simulink model "CodeSysModel"  (R2020b)
settings: Solver=FixedStepAuto  StartTime=0.0  StopTime=inf  FixedStep=2e-2  MaxStep=1e-4  RelTol=1e-3
model workspace (MAT data in the model file):
  sensor_carga = Simulink.Parameter
  sensor_carga.DataType = 'auto'
  sensor_carga.Dimensions = [0 0]
values from neighbouring files (symbols this model uses):
  bcx = 1000e3    (= 1000000)    [Datos_simulacion.m]
  bcy = 500e3    (= 500000)    [Datos_simulacion.m]
  beq_tc = (bv_c+beq_cel)/Rw^2    (= 27000)    [Datos_simulacion.m]
  beq_ti = (b_h+beq_iel)/Rd^2    (= 28800)    [Datos_simulacion.m]
  bw = 30e3    (= 30000)    [Datos_simulacion.m]
  g = 9.80665    [Datos_simulacion.m]
  i_c = 15    [Datos_simulacion.m]
  i_i = 30    [Datos_simulacion.m]
  Kcd = Meq_c*polo_c*n    (= 472500)    [Datos_simulacion.m]
  Kci = Kcp*polo_c/n    (= 1938936.66179)    [Datos_simulacion.m]
  Kcp = Kcd*polo_c    (= 1513396.48861)    [Datos_simulacion.m]
  Kcy = 1.3e9    (= 1300000000)    [Datos_simulacion.m]
  Kid = Kcp*polo_i/n    (= 1815537.84919)    [Datos_simulacion.m]
  Kii = Meq_i*polo_i*n    (= 360000)    [Datos_simulacion.m]
  Kip = Kcd*polo_i    (= 1417080.12441)    [Datos_simulacion.m]
  Kw = 1800e3    (= 1800000)    [Datos_simulacion.m]
  Meq_c = m_c+Jeq_c/Rw^2    (= 59008)    [Datos_simulacion.m]
  Meq_i = m_h+Jeq_i/Rd^2    (= 48014.2222222)    [Datos_simulacion.m]
  Rd = 0.75    [Datos_simulacion.m]
  Rw = 0.5    [Datos_simulacion.m]
  Tau = 1e-3    (= 0.001)    [Datos_simulacion.m]
libraries: simulink x2, fuzblock x1, pid_lib x1, dspswit3 x1
settings Model: PauseTimes=6  Creator=GoniR  LastModifiedBy=GoniR
settings SolverCC: ConcurrentTasks=on  ZeroCrossAlgorithm=Adaptive  AutoInsertRateTranBlk=on
settings DebuggingCC: MaskedZcDiagnostic=none  IgnoredZcDiagnostic=none
settings HardwareCC: ProdHWDeviceType=AMD->x86-64 (Windows64)
settings SFSimCC: SimTargetLang=C++
settings ConfigComp: PLC_TargetIDE=codesys23

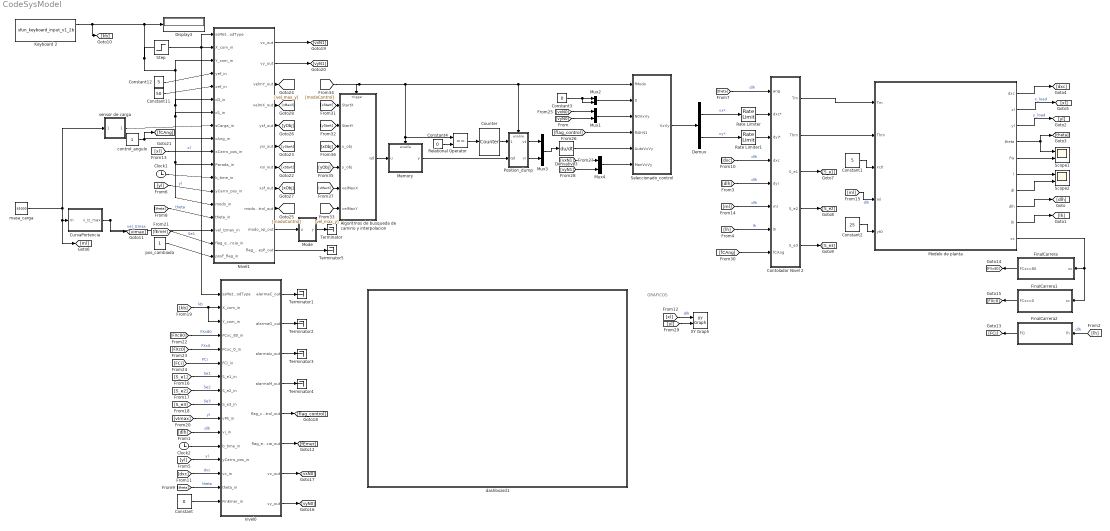
== system CodeSysModel ==
  note: GRAFICOS
  Algoritmos de busqueda de camino y interpolacion : Subsystem
  Clock1 : Clock
  Clock2 : Clock
  Constant : Constant  Value=0
  Constant1 : Constant  Value=5
  Constant11 : Constant  Value=50
  Constant12 : Constant  Value=5
  Constant2 : Constant  Value=25
  Constant3 : Constant  Value=0
  Constant4 : Constant  Value=0
  Contolador Nivel 2 : Subsystem
  Counter : dspswit3/Counter  Direction=Up  CountEvent=Free running  CounterSize=User defined  MaxCount=100000  InitialCount=0  Output=Count  HitValue=32  ResetInput=on  SamplesPerFrame=1  Ts=-1  CntDtype=double  HitDtype=Logical
  CurvaPortencia : MATLAB Function  TreatAsAtomicUnit=on
  Demux : Demux  Outputs=2
  Derivative3 : Derivative
  Display3 : Display
  FinalCarrera : Subsystem
  FinalCarrera1 : Subsystem
  FinalCarrera2 : Subsystem
  Keyboard 2 : M-S-Function  FunctionName=sfun_keyboard_input_v1_2b  mask(Keyboard Input){}
      mask help: Keyboard Input
      mask Display: fprintf('Keyboard');
  Memory : Subsystem
  Mode : MATLAB Function  TreatAsAtomicUnit=on
  Modelo de planta : Subsystem
  Mux{1..4} (4 alike) : Mux  Inputs=2
  Nivel1 : Subsystem  TreatAsAtomicUnit=on  SystemSampleTime=0.02
  Position_dump : Subsystem
  Rate Limiter : RateLimiter  RisingSlewLimit=2  FallingSlewLimit=-2  SampleTimeMode=inherited
  Rate Limiter1 : RateLimiter  RisingSlewLimit=2  FallingSlewLimit=-2  SampleTimeMode=inherited
  Relational Operator : RelationalOperator  Operator===  OutDataTypeStr=boolean  RndMeth=Simplest
  Scope1 : Scope  NumInputPorts=2
  Scope2 : Scope  NumInputPorts=2
  Seleccionado_control : Subsystem
  Step : Step  Time=0.01  SampleTime=0
  Terminator{,1..5} (6 alike) : Terminator
  XY Graph : simulink/Sinks/XY Graph  xmin=0  xmax=80  ymin=0  ymax=60  st=-1
  control_angulo : Constant
  dashboard1 : Subsystem
  masa_carga : Constant  Value=65000
  nivel0 : Subsystem  TreatAsAtomicUnit=on  SystemSampleTime=0.02
  pos_cambiada : Constant
  sensor de carga : Subsystem
  wires:
  Modelo de planta/2(xl) -> [xl]  "x_load"
  Modelo de planta/3(yl) -> [yl]  "y_load"
  Modelo de planta/7(dl) -> Scope2/2
  Modelo de planta/6(l) -> Scope2/1
  Modelo de planta/5(Fw) -> Scope1/2
  masa_carga/1 -> CurvaPortencia/1(m), [ml], sensor de carga/1(In1)
  Constant1/1 -> Modelo de planta/3(xc0)
  Constant2/1 -> Modelo de planta/5(yt0)
  Modelo de planta/4(theta) -> [theta], Scope1/1
  Memory/1(y) -> Position_dump/2(qd)
  Algoritmos de busqueda de camino y interpolacion/1(qd) -> Memory/1(u)
  Position_dump/2(vi) -> Mux3/2
  Demux/2 -> Rate Limiter1/1  "vy*"
  Demux/1 -> Rate Limiter/1  "vx*"
  Nivel1/10(modo_op_out) -> Mode/1(u)
  CurvaPortencia/1(v_Iz_max) -> Nivel1/16(vel_Izmax_in), [vImax]  "vel_Izmax"
  Mode/1(y) -> Terminator/1
  [modoControl] -> Algoritmos de busqueda de camino y interpolacion/Trigger, Relational Operator/1, Memory/Enable, Position_dump/Enable, Seleccionado_control/1(fModo)
  Nivel1/5(ysf_out) -> [yObj]
  Rate Limiter/1 -> Contolador Nivel 2/2(dxc*)
  Modelo de planta/1(dxc) -> [dxc]
  Modelo de planta/8(dlh) -> [dlh]
  Modelo de planta/9(lh) -> [lh]
  Contolador Nivel 2/1(Tm) -> Modelo de planta/1(Tm)
  Contolador Nivel 2/2(Thm) -> Modelo de planta/2(Thm)
  Rate Limiter1/1 -> Contolador Nivel 2/3(dyi*)
  Modelo de planta/10(xc) -> FinalCarrera1/1(xc), FinalCarrera/1(xc)
  Clock2/1 -> nivel0/12(b_time_in)
  nivel0/1(alarmaC_out) -> Terminator1/1
  nivel0/2(alarmaG_out) -> Terminator2/1
  nivel0/3(alarmaIz_out) -> Terminator3/1
  nivel0/4(alarmaM_out) -> Terminator4/1
  Mux3/1 -> Derivative3/1
  Constant/1 -> nivel0/16(FinEmer_in)
  nivel0/6(flag_emergencia_out) -> [fEmer]
  Constant3/1 -> Mux2/1, Mux2/2
  Position_dump/1(vt) -> Mux3/1
  Constant4/1 -> Relational Operator/2
  Relational Operator/1 -> Counter/1
  Counter/1 -> Position_dump/1(counter)
  [dlh] -> Contolador Nivel 2/5(dyi)  "dlh"
  [dlh] -> nivel0/11(vi_in)  "dlh"
  [lh] -> FinalCarrera2/1(lh)  "dlh"
  [lh] -> Contolador Nivel 2/7(lh)  "lh"
  [yl] -> nivel0/13(yCarro_pos_in)  "yl"
  [theta] -> Contolador Nivel 2/1(ang)  "dlh"
  [theta] -> nivel0/15(theta_in)  "theta"
  [dxc] -> Contolador Nivel 2/4(dxc)  "dlh"
  [dxc] -> nivel0/14(vc_in)  "dxc"
  [xl] -> XY Graph/1  "dlh"
  [xl] -> Nivel1/10(xCarro_pos_in)  "xl"
  [ml] -> Contolador Nivel 2/6(ml)  "dlh"
  [ml] -> Modelo de planta/4(ml)  "dlh"
  Contolador Nivel 2/3(S_e1) -> [S_e1]
  Contolador Nivel 2/4(S_e2) -> [S_e2]
  Contolador Nivel 2/5(S_e3) -> [S_e3]
  [S_e1] -> nivel0/7(S_e1_in)  "Se1"
  [S_e2] -> nivel0/8(S_e2_in)  "Se2"
  [S_e3] -> nivel0/9(S_e3_in)  "Se3"
  [kb] -> nivel0/3(Y_com_in), nivel0/2(X_com_in)  "kb"
  [vImax] -> nivel0/10(vMi_in)  "yl"
  FinalCarrera2/1(FCi) -> [FCi]
  FinalCarrera1/1(FCxc<0) -> [FXc0]
  FinalCarrera/1(FCxc>80) -> [FXc80]
  [FCi] -> nivel0/6(FCi_in)  "FCi"
  [FXc0] -> nivel0/5(FCxc_0_in)  "FXc0"
  [FXc80] -> nivel0/4(FCxc_80_in)  "FXc80"
  nivel0/8(vy_out) -> [vyN0]
  nivel0/7(vx_out) -> [vxN0]
  [vyN0] -> Mux1/2
  [vxN0] -> Mux1/1
  nivel0/5(flag_control_out) -> [flag_control]
  Nivel1/1(vx_out) -> [vxN1]
  Nivel1/2(vy_out) -> [vyN1]
  [vxN1] -> Mux4/1
  [vyN1] -> Mux4/2
  Mux2/1 -> Seleccionado_control/2(0)
  Mux1/1 -> Seleccionado_control/3(N0VxVy)
  [flag_control] -> Seleccionado_control/4(fN0-N1)
  Derivative3/1 -> Seleccionado_control/5(AutoVxVy)
  Mux4/1 -> Seleccionado_control/6(ManVxVy)
  Seleccionado_control/1(VxVy) -> Demux/1
  [yl] -> XY Graph/2
  Nivel1/11(flag_disDesP_out) -> Terminator5/1
  [fCAng] -> Contolador Nivel 2/8(fCAng)
  [yl] -> Nivel1/13(yCarro_pos_in)  "yl"
  [theta] -> Nivel1/15(theta_in)  "theta"
  [fEmer] -> Nivel1/17(flag_emergencia_in)  "Se1"
  Keyboard 2/1 -> Display3/1, Nivel1/2(X_com_in), Nivel1/3(Y_com_in), Nivel1/14(modo_in), Nivel1/11(Parada_in), Nivel1/7(cS_in), Nivel1/6(cD_in), [kb]
  Step/1 -> Nivel1/1(ssMethodType), nivel0/1(ssMethodType)
  Constant12/1 -> Nivel1/4(yef_in)
  Constant11/1 -> Nivel1/5(xef_in)
  sensor de carga/1(sCarga_in) -> Nivel1/8(sCarga_in)
  control_angulo/1 -> Nivel1/9(cAng_in), [fCAng]
  Clock1/1 -> Nivel1/12(b_time_in)
  pos_cambiada/1 -> Nivel1/18(posF_flag_in)
  Nivel1/7(xsi_out) -> [xStart]
  [xStart] -> Algoritmos de busqueda de camino y interpolacion/1(StartX)
  Nivel1/6(ysi_out) -> [yStart]
  [yStart] -> Algoritmos de busqueda de camino y interpolacion/2(StartY)
  [vel_max_y] -> Algoritmos de busqueda de camino y interpolacion/6(velMaxY)
  Nivel1/3(velmY_out) -> [vel_max_y]
  Nivel1/9(modo_de_control_out) -> [modoControl]
  [yObj] -> Algoritmos de busqueda de camino y interpolacion/4(y_obj)
  Nivel1/8(xsf_out) -> [xObj]
  [xObj] -> Algoritmos de busqueda de camino y interpolacion/3(x_obj)
  Nivel1/4(velmX_out) -> [vMaxX]
  [vMaxX] -> Algoritmos de busqueda de camino y interpolacion/5(velMaxX)

== system CodeSysModel/Algoritmos de busqueda de camino y interpolacion ==
  StartX : Inport
  StartY : Inport  Port=2
  x_obj : Inport  Port=3
  y_obj : Inport  Port=4
  velMaxX : Inport  Port=5
  velMaxY : Inport  Port=6
  Trigger : TriggerPort  VariantControl=Variant  PortDimensions=1
  Astart : MATLAB Function  TreatAsAtomicUnit=on
  Interpolador : MATLAB Function  TreatAsAtomicUnit=on
  qd : Outport
  wires:
  StartX/1 -> Astart/1(StartX)
  y_obj/1 -> Astart/4(y_obj)
  x_obj/1 -> Astart/3(x_obj)
  StartY/1 -> Astart/2(StartY)
  Astart/1(OptimalPath2) -> Interpolador/1(wayPoints)
  velMaxX/1 -> Interpolador/2(velMaxX)
  velMaxY/1 -> Interpolador/3(velMaxY)
  Interpolador/1(q) -> qd/1

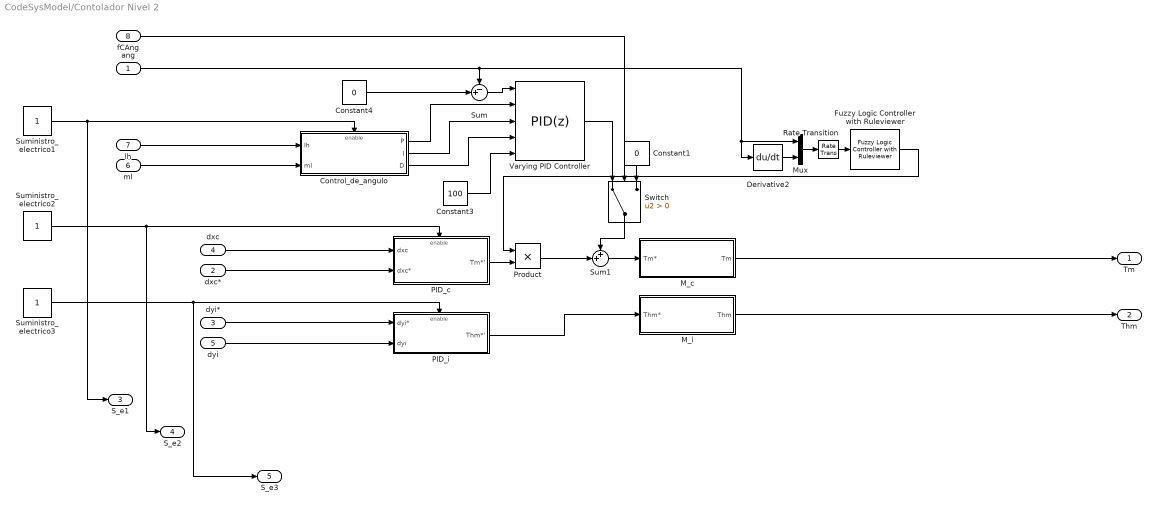
== system CodeSysModel/Contolador Nivel 2 ==
  ang : Inport
  dxc* : Inport  Port=2
  dyi* : Inport  Port=3
  dxc : Inport  Port=4
  dyi : Inport  Port=5
  ml : Inport  Port=6
  lh : Inport  Port=7
  fCAng : Inport  Port=8
  Constant1 : Constant  Value=0
  Constant3 : Constant  Value=100
  Constant4 : Constant  Value=0
  Control_de_angulo : Subsystem
  Derivative2 : Derivative
  Fuzzy Logic Controller with Ruleviewer : fuzblock/Fuzzy Logic  Controller  with Ruleviewer  fismatrix=Control2  Ts=0.5
  M_c : Subsystem
  M_i : Subsystem
  Mux : Mux  Inputs=2
  PID_c : Subsystem
  PID_i : Subsystem
  Product : Product
  Rate Transition : RateTransition  OutPortSampleTime=0.02
  Sum : Sum  Inputs=-+|
  Sum1 : Sum  Inputs=++|
  Suministro_electrico1 : Constant
  Suministro_electrico2 : Constant
  Suministro_electrico3 : Constant
  Switch : Switch  Criteria=u2 > Threshold
  Varying PID Controller : pid_lib/PID Controller  Controller=PID  Form=Parallel  TimeDomain=Discrete-time  UseExternalTs=off  SampleTime=0.02  IntegratorMethod=Forward Euler  FilterMethod=Forward Euler  ControllerParametersSource=external  P=1  I=1  D=0  UseFilter=on  N=100  TunerSelectOption=Transfer Function Based (PID Tuner App)  InitialConditionSource=internal  InitialConditionForIntegrator=0  InitialConditionForFilter=0  DifferentiatorICPrevScaledInput=0  ExternalReset=none  TrackingMode=off  Kt=1  LimitOutput=off  SatLimitsSource=internal  UpperSaturationLimit=inf  LowerSaturationLimit=-inf  LinearizeAsGain=on  AntiWindupMode=none  Kb=1  POutMin=[]  POutMax=[]  IOutMin=[]  IOutMax=[]  DOutMin=[]  DOutMax=[]  NOutMin=[]  NOutMax=[]  SumOutMin=[]  SumOutMax=[]  SaturationOutMin=[]  SaturationOutMax=[]  PParamMin=[]  PParamMax=[]  IParamMin=[]  IParamMax=[]  DParamMin=[]  DParamMax=[]  NParamMin=[]  NParamMax=[]  KbParamMin=[]  KbParamMax=[]  KtParamMin=[]  KtParamMax=[]  KbOutMin=[]  KbOutMax=[]  KtOutMin=[]  KtOutMax=[]  IntegratorOutMin=[]  IntegratorOutMax=[]  FilterOutMin=[]  FilterOutMax=[]  SumI1OutMin=[]  SumI1OutMax=[]  SumI2OutMin=[]  SumI2OutMax=[]  SumI3OutMin=[]  SumI3OutMax=[]  SumI4OutMin=[]  SumI4OutMax=[]  SumDOutMin=[]  SumDOutMax=[]  DifferentiatorOutMin=[]  DifferentiatorOutMax=[]  FilterDiffOutCoefMin=[]  FilterDiffOutCoefMax=[]  ReciprocalOutMin=[]  ReciprocalOutMax=[]  SumDenOutMin=[]  SumDenOutMax=[]  SumNumOutMin=[]  SumNumOutMax=[]  DivideOutMin=[]  DivideOutMax=[]  UdiffTsProdOutMin=[]  UdiffTsProdOutMax=[]  NTsProdOutMin=[]  NTsProdOutMax=[]  UintegralTsProdOutMin=[]  UintegralTsProdOutMax=[]  UngainTsProdOutMin=[]  UngainTsProdOutMax=[]  IntegratorContinuousStateAttributes=''  IntegratorStateMustResolveToSignalObject=off  IntegratorRTWStateStorageClass=Auto  FilterContinuousStateAttributes=''  FilterStateMustResolveToSignalObject=off  FilterRTWStateStorageClass=Auto  ParallelPVariant=ExternalParameters  IdealPVariant=Disabled  IVariant=ExternalParameters  DVariant=ExternalParameters  IntegratorVariant=Discrete  SatVariant=Disabled  AWVariant=Passthrough  PCopyVariant=Disabled  TRVariant=Disabled  FdbkBlocksVariant=Forward  IdealPFdbkVariant=Disabled  SatFdbkVariant=Disabled  DerivativeFilterVariant=ForwardEulerFilter  NVariant=ExternalParameters  NCopyVariant=Disabled  FilterICVariant=InternalICsFilter  IntegratorICVariant=InternalICs  ExternalResetVariant=Disabled  TRSumVariant=Passthrough  SumFdbkVariant=Disabled  SumVariant=Sum_PID  TsampFilterVariant=InternalTs  TsampNgainVariant=Passthrough  TsampIntegralVariant=Passthrough  ExternalSaturationOutDataTypeStr=Inherit: Same as second input
  Tm : Outport
  Thm : Outport  Port=2
  S_e1 : Outport  Port=3
  S_e2 : Outport  Port=4
  S_e3 : Outport  Port=5
  wires:
  Constant3/1 -> Varying PID Controller/5
  Fuzzy Logic Controller with Ruleviewer/1 -> Product/1
  Rate Transition/1 -> Fuzzy Logic Controller with Ruleviewer/1
  M_i/1(Thm) -> Thm/1
  ang/1 -> Derivative2/1, Mux/1, Sum/1
  Constant4/1 -> Sum/2
  Control_de_angulo/1(P) -> Varying PID Controller/2
  PID_i/1(Thm*') -> M_i/1(Thm*)
  Sum/1 -> Varying PID Controller/1
  Control_de_angulo/3(D) -> Varying PID Controller/4
  Product/1 -> Sum1/2
  Control_de_angulo/2(I) -> Varying PID Controller/3
  ml/1 -> Control_de_angulo/2(ml)
  Mux/1 -> Rate Transition/1
  PID_c/1(Tm*') -> Product/2
  Sum1/1 -> M_c/1(Tm*)
  M_c/1(Tm) -> Tm/1
  dxc*/1 -> PID_c/2(dxc*)
  lh/1 -> Control_de_angulo/1(lh)
  dyi*/1 -> PID_i/1(dyi*)
  dxc/1 -> PID_c/1(dxc)
  dyi/1 -> PID_i/2(dyi)
  Derivative2/1 -> Mux/2
  Suministro_electrico1/1 -> S_e1/1, Control_de_angulo/Enable
  Suministro_electrico3/1 -> PID_i/Enable, S_e3/1
  Suministro_electrico2/1 -> S_e2/1, PID_c/Enable
  Switch/1 -> Sum1/1
  fCAng/1 -> Switch/2
  Constant1/1 -> Switch/3
  Varying PID Controller/1 -> Switch/1

== system CodeSysModel/FinalCarrera ==
  xc : Inport
  Constant : Constant
  Constant1 : Constant  Value=0
  Switch : Switch  Criteria=u2 > Threshold  Threshold=80
  FCxc>80 : Outport
  wires:
  Constant/1 -> Switch/1
  Constant1/1 -> Switch/3
  Switch/1 -> FCxc>80/1
  xc/1 -> Switch/2

== system CodeSysModel/FinalCarrera1 ==
  xc : Inport
  Constant : Constant
  Constant1 : Constant  Value=0
  Gain : Gain  Gain=-1
  Switch : Switch  Criteria=u2 > Threshold
  FCxc<0 : Outport
  wires:
  Constant/1 -> Switch/1
  Constant1/1 -> Switch/3
  Switch/1 -> FCxc<0/1
  xc/1 -> Gain/1
  Gain/1 -> Switch/2

== system CodeSysModel/FinalCarrera2 ==
  lh : Inport
  Constant : Constant
  Constant1 : Constant  Value=0
  Gain : Gain  Gain=-1
  Switch : Switch
  FCi : Outport
  wires:
  Constant/1 -> Switch/1
  Constant1/1 -> Switch/3
  Switch/1 -> FCi/1
  lh/1 -> Gain/1
  Gain/1 -> Switch/2

== system CodeSysModel/Memory ==
  u : Inport
  Enable : EnablePort
  y : Outport
  wires:
  u/1 -> y/1

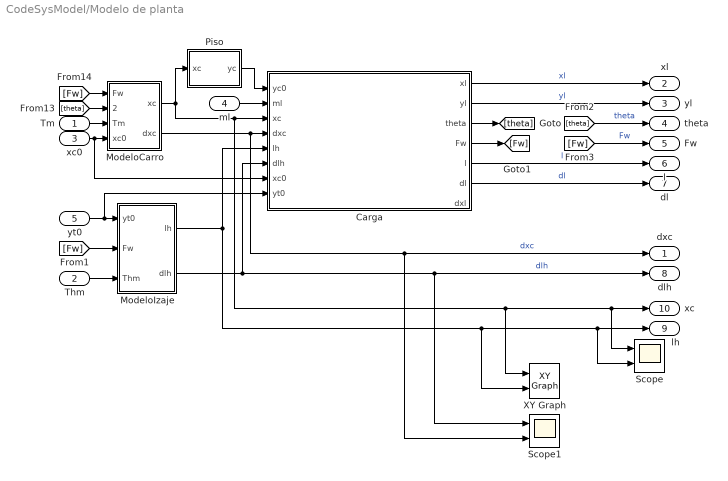
== system CodeSysModel/Modelo de planta ==
  Tm : Inport
  Thm : Inport  Port=2
  xc0 : Inport  Port=3
  ml : Inport  Port=4
  yt0 : Inport  Port=5
  Carga : Subsystem
  ModeloCarro : Subsystem
  ModeloIzaje : Subsystem
  Piso : Subsystem
  Scope : Scope  NumInputPorts=2
  Scope1 : Scope  NumInputPorts=2
  XY Graph : simulink/Sinks/XY Graph  xmin=0  xmax=80  ymin=0  ymax=60  st=-1
  dxc : Outport
  xl : Outport  Port=2
  yl : Outport  Port=3
  theta : Outport  Port=4
  Fw : Outport  Port=5
  l : Outport  Port=6
  dl : Outport  Port=7
  dlh : Outport  Port=8
  lh : Outport  Port=9
  xc : Outport  Port=10
  wires:
  ModeloCarro/1(xc) -> XY Graph/1, Scope/1, xc/1, Carga/3(xc), Piso/1(xc)
  ModeloCarro/2(dxc) -> Scope1/2, dxc/1, Carga/4(dxc)  "dxc"
  ModeloIzaje/1(lh) -> XY Graph/2, Scope/2, lh/1, Carga/5(lh)
  ModeloIzaje/2(dlh) -> Carga/6(dlh), Scope1/1, dlh/1  "dlh"
  Carga/4(Fw) -> [Fw]
  [Fw] -> ModeloCarro/1(Fw)
  [Fw] -> ModeloIzaje/2(Fw)
  Carga/3(theta) -> [theta]
  [theta] -> ModeloCarro/2(theta)
  Carga/1(xl) -> xl/1  "xl"
  Carga/2(yl) -> yl/1  "yl"
  Carga/5(l) -> l/1  "l"
  Carga/6(dl) -> dl/1  "dl"
  [theta] -> theta/1  "theta"
  [Fw] -> Fw/1  "Fw"
  ml/1 -> Carga/2(ml)
  Thm/1 -> ModeloIzaje/3(Thm)
  Tm/1 -> ModeloCarro/3(Tm)
  Piso/1(yc) -> Carga/1(yc0)
  yt0/1 -> Carga/8(yt0), ModeloIzaje/1(yt0)
  xc0/1 -> Carga/7(xc0), ModeloCarro/4(xc0)

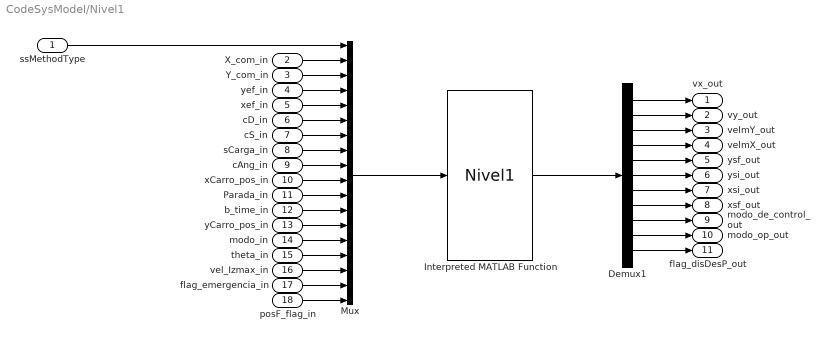
== system CodeSysModel/Nivel1 ==
  ssMethodType : Inport
  X_com_in : Inport  Port=2
  Y_com_in : Inport  Port=3
  yef_in : Inport  Port=4
  xef_in : Inport  Port=5
  cD_in : Inport  Port=6
  cS_in : Inport  Port=7
  sCarga_in : Inport  Port=8
  cAng_in : Inport  Port=9
  xCarro_pos_in : Inport  Port=10
  Parada_in : Inport  Port=11
  b_time_in : Inport  Port=12
  yCarro_pos_in : Inport  Port=13
  modo_in : Inport  Port=14
  theta_in : Inport  Port=15
  vel_Izmax_in : Inport  Port=16
  flag_emergencia_in : Inport  Port=17
  posF_flag_in : Inport  Port=18
  Demux1 : Demux  Outputs=11
  Interpreted MATLAB Function : MATLABFcn  MATLABFcn=Nivel1  OutputDimensions=11  Output1D=off
  Mux : Mux  Inputs=18
  vx_out : Outport
  vy_out : Outport  Port=2
  velmY_out : Outport  Port=3
  velmX_out : Outport  Port=4
  ysf_out : Outport  Port=5
  ysi_out : Outport  Port=6
  xsi_out : Outport  Port=7
  xsf_out : Outport  Port=8
  modo_de_control_out : Outport  Port=9
  modo_op_out : Outport  Port=10
  flag_disDesP_out : Outport  Port=11
  wires:
  Interpreted MATLAB Function/1 -> Demux1/1
  ssMethodType/1 -> Mux/1
  X_com_in/1 -> Mux/2
  Y_com_in/1 -> Mux/3
  yef_in/1 -> Mux/4
  xef_in/1 -> Mux/5
  cD_in/1 -> Mux/6
  cS_in/1 -> Mux/7
  sCarga_in/1 -> Mux/8
  cAng_in/1 -> Mux/9
  xCarro_pos_in/1 -> Mux/10
  Parada_in/1 -> Mux/11
  b_time_in/1 -> Mux/12
  yCarro_pos_in/1 -> Mux/13
  modo_in/1 -> Mux/14
  theta_in/1 -> Mux/15
  vel_Izmax_in/1 -> Mux/16
  flag_emergencia_in/1 -> Mux/17
  posF_flag_in/1 -> Mux/18
  Demux1/1 -> vx_out/1
  Demux1/2 -> vy_out/1
  Demux1/3 -> velmY_out/1
  Demux1/4 -> velmX_out/1
  Demux1/5 -> ysf_out/1
  Demux1/6 -> ysi_out/1
  Demux1/7 -> xsi_out/1
  Demux1/8 -> xsf_out/1
  Demux1/9 -> modo_de_control_out/1
  Demux1/10 -> modo_op_out/1
  Demux1/11 -> flag_disDesP_out/1
  Mux/1 -> Interpreted MATLAB Function/1

== system CodeSysModel/Position_dump ==
  counter : Inport
  qd : Inport  Port=2
  Enable : EnablePort  PropagateVarSize=During execution
  MATLAB Function : MATLAB Function  TreatAsAtomicUnit=on
  Rate Transition : RateTransition
  Scope1 : Scope
  vt : Outport
  vi : Outport  Port=2
  wires:
  MATLAB Function/1(vt) -> vt/1
  MATLAB Function/2(vi) -> vi/1
  qd/1 -> MATLAB Function/1(qd)
  Rate Transition/1 -> Scope1/1, MATLAB Function/2(cont_i)
  counter/1 -> Rate Transition/1

== system CodeSysModel/Seleccionado_control ==
  fModo : Inport
  0 : Inport  Port=2
  N0VxVy : Inport  Port=3
  fN0-N1 : Inport  Port=4
  AutoVxVy : Inport  Port=5
  ManVxVy : Inport  Port=6
  AutoOn/Off : Switch  Criteria=u2 > Threshold
  M_o_A : Switch  Criteria=u2 > Threshold
  N0_o_N1 : Switch  Criteria=u2 > Threshold
  VxVy : Outport
  wires:
  AutoOn/Off/1 -> M_o_A/1
  N0_o_N1/1 -> VxVy/1
  M_o_A/1 -> N0_o_N1/3
  ManVxVy/1 -> M_o_A/3
  AutoVxVy/1 -> AutoOn/Off/1
  fModo/1 -> AutoOn/Off/2, M_o_A/2
  0/1 -> AutoOn/Off/3
  fN0-N1/1 -> N0_o_N1/2
  N0VxVy/1 -> N0_o_N1/1

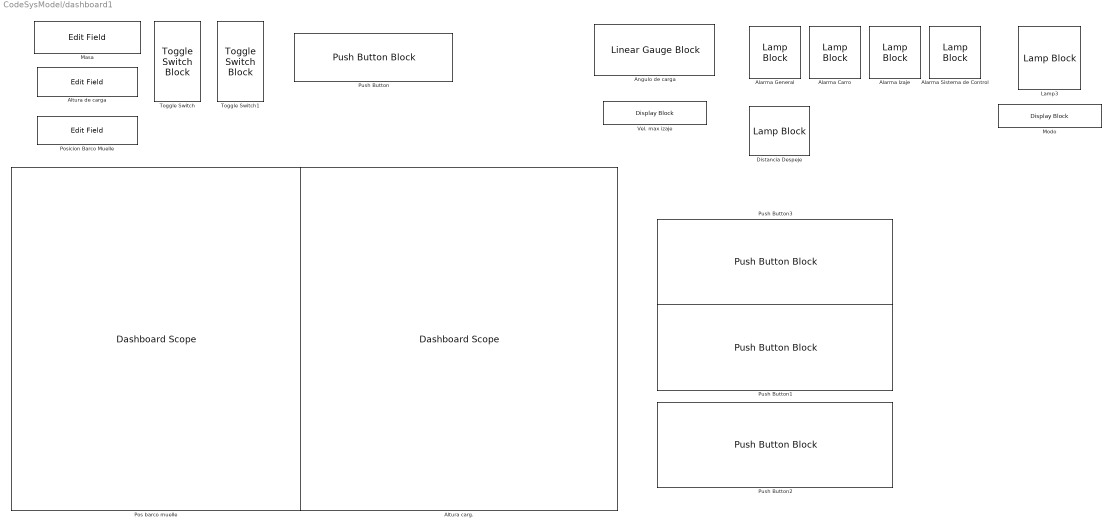
== system CodeSysModel/dashboard1 ==
  Alarma Carro : LampBlock
  Alarma General : LampBlock
  Alarma Izaje : LampBlock
  Alarma Sistema de Control : LampBlock
  Altura carg. : DashboardScope
  Altura de carga : EditField  LabelPosition=Hide  ShowInitialText=on  Alignment=Center
  Angulo de carga : LinearGaugeBlock  LabelPosition=Hide  ScaleMin=-0.15  ScaleMax=0.15
  Distancia Despeje : LampBlock
  Lamp3 : LampBlock  LabelPosition=Bottom
  Masa : EditField  LabelPosition=Hide  ShowInitialText=on  Alignment=Center
  Modo : DisplayBlock  LabelPosition=Hide  Format=short  Transparency=1
  Pos barco muelle : DashboardScope
  Posicion Barco Muelle : EditField  LabelPosition=Hide  ShowInitialText=on  Alignment=Center
  Push Button : PushButtonBlock  ButtonText=Fin Emergencia
  Push Button1 : PushButtonBlock  ButtonText=Falla Microcontrolador1  OnValue=0
  Push Button2 : PushButtonBlock  ButtonText=Falla Microcontrolador3  OnValue=0
  Push Button3 : PushButtonBlock  ButtonText=Falla Microcontrolador2  OnValue=0
  Toggle Switch : ToggleSwitchBlock
      settings: Values={{'Off', 'On'}, [0 1]}
  Toggle Switch1 : ToggleSwitchBlock
      settings: Values={{'Sin Cambiar', 'Cambiada'}, [0 1]}
  Vel. max izaje : DisplayBlock  LabelPosition=Hide  Format=short  Transparency=1

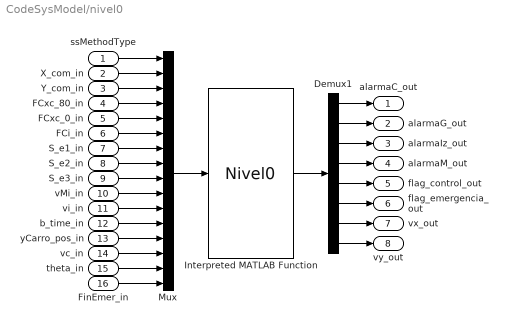
== system CodeSysModel/nivel0 ==
  ssMethodType : Inport
  X_com_in : Inport  Port=2
  Y_com_in : Inport  Port=3
  FCxc_80_in : Inport  Port=4
  FCxc_0_in : Inport  Port=5
  FCi_in : Inport  Port=6
  S_e1_in : Inport  Port=7
  S_e2_in : Inport  Port=8
  S_e3_in : Inport  Port=9
  vMi_in : Inport  Port=10
  vi_in : Inport  Port=11
  b_time_in : Inport  Port=12
  yCarro_pos_in : Inport  Port=13
  vc_in : Inport  Port=14
  theta_in : Inport  Port=15
  FinEmer_in : Inport  Port=16
  Demux1 : Demux  Outputs=8
  Interpreted MATLAB Function : MATLABFcn  MATLABFcn=Nivel0  OutputDimensions=8  Output1D=off
  Mux : Mux  Inputs=16
  alarmaC_out : Outport
  alarmaG_out : Outport  Port=2
  alarmaIz_out : Outport  Port=3
  alarmaM_out : Outport  Port=4
  flag_control_out : Outport  Port=5
  flag_emergencia_out : Outport  Port=6
  vx_out : Outport  Port=7
  vy_out : Outport  Port=8
  wires:
  Interpreted MATLAB Function/1 -> Demux1/1
  ssMethodType/1 -> Mux/1
  X_com_in/1 -> Mux/2
  Y_com_in/1 -> Mux/3
  FCxc_80_in/1 -> Mux/4
  FCxc_0_in/1 -> Mux/5
  FCi_in/1 -> Mux/6
  S_e1_in/1 -> Mux/7
  S_e2_in/1 -> Mux/8
  S_e3_in/1 -> Mux/9
  vMi_in/1 -> Mux/10
  vi_in/1 -> Mux/11
  b_time_in/1 -> Mux/12
  yCarro_pos_in/1 -> Mux/13
  vc_in/1 -> Mux/14
  theta_in/1 -> Mux/15
  FinEmer_in/1 -> Mux/16
  Demux1/1 -> alarmaC_out/1
  Demux1/2 -> alarmaG_out/1
  Demux1/3 -> alarmaIz_out/1
  Demux1/4 -> alarmaM_out/1
  Demux1/5 -> flag_control_out/1
  Demux1/6 -> flag_emergencia_out/1
  Demux1/7 -> vx_out/1
  Demux1/8 -> vy_out/1
  Mux/1 -> Interpreted MATLAB Function/1

== system CodeSysModel/sensor de carga ==
  In1 : Inport
  Constant5 : Constant
  Constant6 : Constant  Value=0
  Switch1 : Switch  Criteria=u2 > Threshold  Threshold=15000
  sCarga_in : Outport
  wires:
  Constant5/1 -> Switch1/1
  Constant6/1 -> Switch1/3
  Switch1/1 -> sCarga_in/1
  In1/1 -> Switch1/2

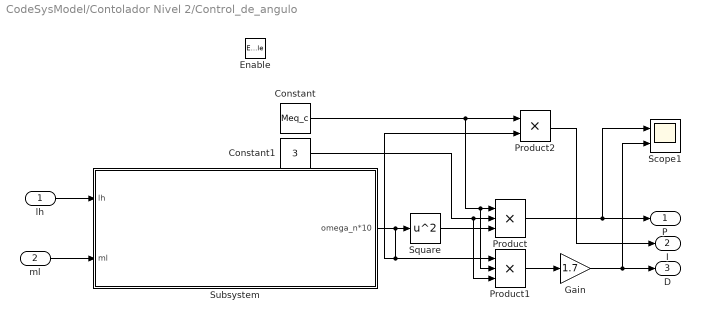
== system CodeSysModel/Contolador Nivel 2/Control_de_angulo ==
  lh : Inport
  ml : Inport  Port=2
  Enable : EnablePort
  Constant : Constant  Value=Meq_c
  Constant1 : Constant  Value=3
  Gain : Gain  Gain=1.7
  Product : Product  Inputs=3
  Product1 : Product  Inputs=3
  Product2 : Product
  Scope1 : Scope  NumInputPorts=2
  Square : Math  Operator=square  SaturateOnIntegerOverflow=on
  Subsystem : Subsystem
  P : Outport
  I : Outport  Port=2
  D : Outport  Port=3
  wires:
  lh/1 -> Subsystem/1(lh)
  Constant1/1 -> Product/2, Product1/3
  Subsystem/1(omega_n*10) -> Product1/1, Product2/2, Square/1
  Constant/1 -> Product1/2, Product/1, Product2/1
  Product/1 -> P/1, Scope1/1
  Product1/1 -> Gain/1
  Square/1 -> Product/3
  ml/1 -> Subsystem/2(ml)
  Product2/1 -> I/1
  Gain/1 -> D/1, Scope1/2

== system CodeSysModel/Contolador Nivel 2/M_c ==
  Tm* : Inport
  Transfer Fcn : TransferFcn  Denominator=[Tau 1]
  Tm : Outport
  wires:
  Tm*/1 -> Transfer Fcn/1
  Transfer Fcn/1 -> Tm/1

== system CodeSysModel/Contolador Nivel 2/M_i ==
  Thm* : Inport
  Transfer Fcn : TransferFcn  Denominator=[Tau 1]
  Thm : Outport
  wires:
  Thm*/1 -> Transfer Fcn/1
  Transfer Fcn/1 -> Thm/1

== system CodeSysModel/Contolador Nivel 2/PID_c ==
  dxc : Inport
  dxc* : Inport  Port=2
  Enable : EnablePort
  Gain : Gain  Gain=Kcp
  Gain1 : Gain  Gain=Kci
  Gain2 : Gain  Gain=Kcd
  Integrator : Integrator
  Integrator1 : Integrator
  Sum : Sum  Inputs=|+-
  Sum1 : Sum  Inputs=+++
  Tm*' : Outport
  wires:
  dxc*/1 -> Sum/1
  dxc/1 -> Sum/2
  Sum1/1 -> Tm*'/1
  Gain2/1 -> Sum1/3
  Gain/1 -> Sum1/2
  Gain1/1 -> Sum1/1
  Sum/1 -> Integrator1/1, Gain2/1
  Integrator1/1 -> Integrator/1, Gain/1
  Integrator/1 -> Gain1/1

== system CodeSysModel/Contolador Nivel 2/PID_i ==
  dyi* : Inport
  dyi : Inport  Port=2
  Enable : EnablePort
  Gain : Gain  Gain=Kip
  Gain1 : Gain  Gain=Kii
  Gain2 : Gain  Gain=Kid
  Integrator : Integrator
  Integrator1 : Integrator
  Sum : Sum  Inputs=|+-
  Sum1 : Sum  Inputs=+++
  Thm*' : Outport
  wires:
  dyi*/1 -> Sum/1
  dyi/1 -> Sum/2
  Sum1/1 -> Thm*'/1
  Gain2/1 -> Sum1/3
  Gain/1 -> Sum1/2
  Gain1/1 -> Sum1/1
  Sum/1 -> Integrator/1, Gain2/1
  Integrator/1 -> Integrator1/1, Gain/1
  Integrator1/1 -> Gain1/1

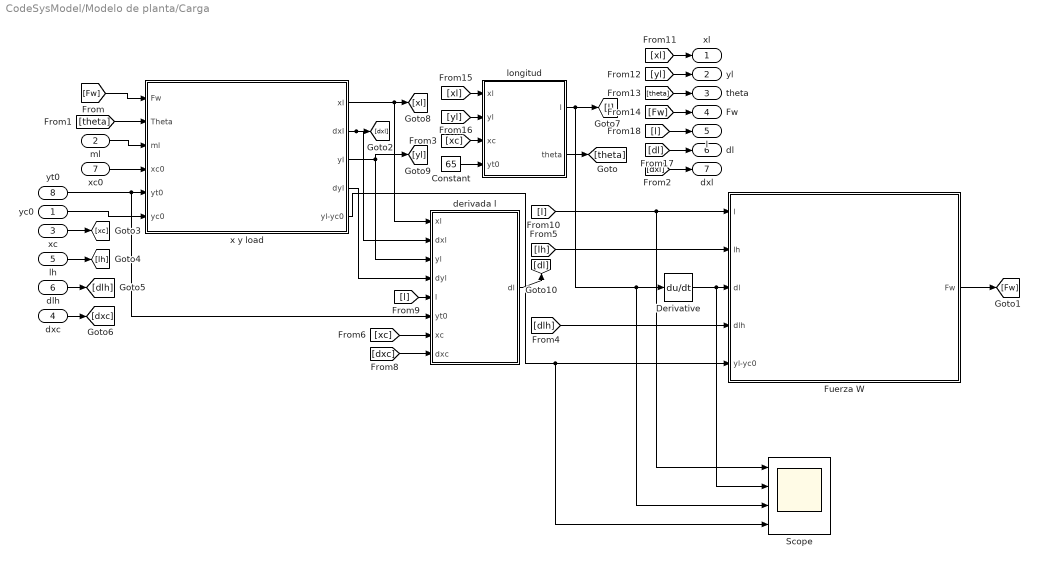
== system CodeSysModel/Modelo de planta/Carga ==
  yc0 : Inport
  ml : Inport  Port=2
  xc : Inport  Port=3
  dxc : Inport  Port=4
  lh : Inport  Port=5
  dlh : Inport  Port=6
  xc0 : Inport  Port=7
  yt0 : Inport  Port=8
  Constant : Constant  Value=65
  Derivative : Derivative
  Fuerza W : Subsystem
  Scope : Scope  NumInputPorts=4
  derivada l : Subsystem
  longitud : Subsystem
  x y load : Subsystem
  xl : Outport
  yl : Outport  Port=2
  theta : Outport  Port=3
  Fw : Outport  Port=4
  l : Outport  Port=5
  dl : Outport  Port=6
  dxl : Outport  Port=7
  wires:
  x y load/3(yl) -> [yl], derivada l/3(yl)
  derivada l/1(dl) -> [dl]
  longitud/2(theta) -> [theta]
  Fuerza W/1(Fw) -> [Fw]
  [theta] -> x y load/2(Theta)
  [Fw] -> x y load/1(Fw)
  ml/1 -> x y load/3(ml)
  yc0/1 -> x y load/6(yc0)
  xc/1 -> [xc]
  [xc] -> longitud/3(xc)
  lh/1 -> [lh]
  dlh/1 -> [dlh]
  [lh] -> Fuerza W/2(lh)
  [dlh] -> Fuerza W/4(dlh)
  x y load/1(xl) -> [xl], derivada l/1(xl)
  x y load/2(dxl) -> derivada l/2(dxl), [dxl]
  x y load/4(dyl) -> derivada l/4(dyl)
  dxc/1 -> [dxc]
  longitud/1(l) -> Scope/3, Derivative/1, [l]
  [l] -> Fuerza W/1(l), Scope/1
  [xl] -> xl/1
  [yl] -> yl/1
  [theta] -> theta/1
  [Fw] -> Fw/1
  [xl] -> longitud/1(xl)
  [yl] -> longitud/2(yl)
  [dl] -> dl/1
  [l] -> l/1
  [l] -> derivada l/5(l)
  [xc] -> derivada l/7(xc)
  [dxc] -> derivada l/8(dxc)
  x y load/5(yl-yc0) -> Scope/4, Fuerza W/5(yl-yc0)
  xc0/1 -> x y load/4(xc0)
  [dxl] -> dxl/1
  Constant/1 -> longitud/4(yt0)
  yt0/1 -> derivada l/6(yt0), x y load/5(yt0)
  Derivative/1 -> Scope/2, Fuerza W/3(dl)

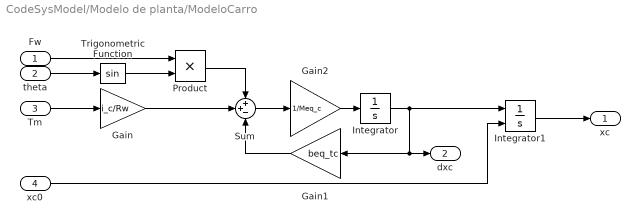
== system CodeSysModel/Modelo de planta/ModeloCarro ==
  Fw : Inport
  theta : Inport  Port=2
  Tm : Inport  Port=3
  xc0 : Inport  Port=4
  Gain : Gain  Gain=i_c/Rw
  Gain1 : Gain  Gain=beq_tc
  Gain2 : Gain  Gain=1/Meq_c
  Integrator : Integrator
  Integrator1 : Integrator  InitialConditionSource=external  InitialCondition=0.01
  Product : Product
  Sum : Sum  Inputs=++-
  Trigonometric Function : Trigonometry
  xc : Outport
  dxc : Outport  Port=2
  wires:
  Product/1 -> Sum/1
  Integrator1/1 -> xc/1
  Gain2/1 -> Integrator/1
  Fw/1 -> Product/1
  Gain1/1 -> Sum/3
  Integrator/1 -> Integrator1/1, dxc/1, Gain1/1
  Tm/1 -> Gain/1
  Trigonometric Function/1 -> Product/2
  Sum/1 -> Gain2/1
  theta/1 -> Trigonometric Function/1
  Gain/1 -> Sum/2
  xc0/1 -> Integrator1/2

== system CodeSysModel/Modelo de planta/ModeloIzaje ==
  yt0 : Inport
  Fw : Inport  Port=2
  Thm : Inport  Port=3
  Constant : Constant  Value=65
  Gain : Gain  Gain=+i_i/Rd
  Gain1 : Gain  Gain=beq_ti
  Gain2 : Gain  Gain=1/Meq_i
  Integrator : Integrator
  Integrator1 : Integrator  InitialConditionSource=external  InitialCondition=0.5
  Sum : Sum  Inputs=++-
  Sum1 : Sum  Inputs=|-+
  lh : Outport
  dlh : Outport  Port=2
  wires:
  Fw/1 -> Sum/1
  Integrator1/1 -> lh/1
  Gain2/1 -> Integrator/1
  Gain1/1 -> Sum/3
  Integrator/1 -> Integrator1/1, Gain1/1, dlh/1
  Thm/1 -> Gain/1
  Sum/1 -> Gain2/1
  Gain/1 -> Sum/2
  Sum1/1 -> Integrator1/2
  yt0/1 -> Sum1/1
  Constant/1 -> Sum1/2

== system CodeSysModel/Modelo de planta/Piso ==
  xc : Inport
  Constant : Constant  Value=0
  yc : Outport
  wires:
  Constant/1 -> yc/1

== system CodeSysModel/Contolador Nivel 2/Control_de_angulo/Subsystem ==
  lh : Inport
  ml : Inport  Port=2
  Constant : Constant  Value=g
  Constant1 : Constant  Value=Meq_c
  Divide1 : Product  Inputs=*//
  Gain : Gain  Gain=10
  Gain1 : Gain  Gain=Meq_c
  Scope : Scope
  Scope1 : Scope
  Sqrt : Sqrt  SaturateOnIntegerOverflow=on
  Sum : Sum  Inputs=|++
  omega_n*10 : Outport
  wires:
  Sqrt/1 -> Scope1/1, Gain/1
  lh/1 -> Scope/1, Divide1/2
  Divide1/1 -> Sqrt/1
  Constant/1 -> Gain1/1
  Gain1/1 -> Divide1/1
  ml/1 -> Sum/1
  Constant1/1 -> Sum/2
  Sum/1 -> Divide1/3
  Gain/1 -> omega_n*10/1

== system CodeSysModel/Modelo de planta/Carga/Fuerza W ==
  l : Inport
  lh : Inport  Port=2
  dl : Inport  Port=3
  dlh : Inport  Port=4
  yl-yc0 : Inport  Port=5
  Gain : Gain  Gain=Kw
  Gain1 : Gain  Gain=0
  Gain2 : Gain  Gain=bw
  Sum : Sum  Inputs=|+-
  Sum1 : Sum  Inputs=|+-
  Sum2 : Sum  Inputs=|++
  Switch : Switch  Criteria=u2 > Threshold
  Fw : Outport
  wires:
  yl-yc0/1 -> Switch/2
  l/1 -> Sum/1
  lh/1 -> Sum/2
  Sum/1 -> Gain1/1, Gain/1
  Gain/1 -> Switch/1
  Gain1/1 -> Switch/3
  dl/1 -> Sum1/1
  dlh/1 -> Sum1/2
  Sum1/1 -> Gain2/1
  Switch/1 -> Sum2/1
  Gain2/1 -> Sum2/2
  Sum2/1 -> Fw/1

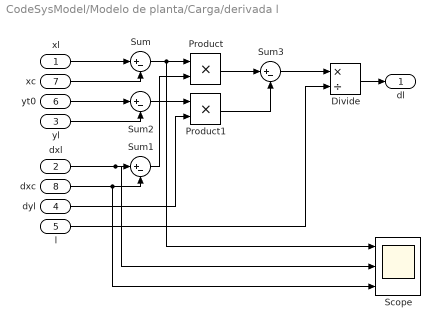
== system CodeSysModel/Modelo de planta/Carga/derivada l ==
  xl : Inport
  dxl : Inport  Port=2
  yl : Inport  Port=3
  dyl : Inport  Port=4
  l : Inport  Port=5
  yt0 : Inport  Port=6
  xc : Inport  Port=7
  dxc : Inport  Port=8
  Divide : Product  Inputs=*/
  Product : Product
  Product1 : Product
  Scope : Scope  NumInputPorts=3
  Sum{,1..3} (4 alike) : Sum  Inputs=|+-
  dl : Outport
  wires:
  xl/1 -> Sum/1
  xc/1 -> Sum/2
  dxl/1 -> Scope/2, Sum1/1
  dxc/1 -> Scope/3, Sum1/2
  Sum/1 -> Scope/1, Product/1
  Sum1/1 -> Product/2
  yt0/1 -> Sum2/1
  yl/1 -> Sum2/2
  dyl/1 -> Product1/2
  Sum2/1 -> Product1/1
  Product/1 -> Sum3/1
  Product1/1 -> Sum3/2
  Sum3/1 -> Divide/1
  Divide/1 -> dl/1
  l/1 -> Divide/2

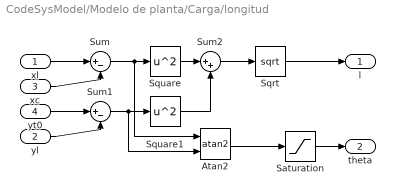
== system CodeSysModel/Modelo de planta/Carga/longitud ==
  xl : Inport
  yl : Inport  Port=2
  xc : Inport  Port=3
  yt0 : Inport  Port=4
  Atan2 : Trigonometry  Operator=atan2
  Saturation : Saturate  UpperLimit=pi/2  LowerLimit=-pi/2
  Sqrt : Sqrt  OutputSignalType=real  SaturateOnIntegerOverflow=on
  Square : Math  Operator=square  OutputSignalType=real  SaturateOnIntegerOverflow=on
  Square1 : Math  Operator=square  OutputSignalType=real  SaturateOnIntegerOverflow=on
  Sum : Sum  Inputs=|+-
  Sum1 : Sum  Inputs=|+-
  Sum2 : Sum  Inputs=|++
  l : Outport
  theta : Outport  Port=2
  wires:
  xl/1 -> Sum/1
  xc/1 -> Sum/2
  Sum/1 -> Atan2/1, Square/1
  yt0/1 -> Sum1/1
  yl/1 -> Sum1/2
  Sum1/1 -> Atan2/2, Square1/1
  Square/1 -> Sum2/1
  Square1/1 -> Sum2/2
  Sum2/1 -> Sqrt/1
  Atan2/1 -> Saturation/1
  Saturation/1 -> theta/1
  Sqrt/1 -> l/1

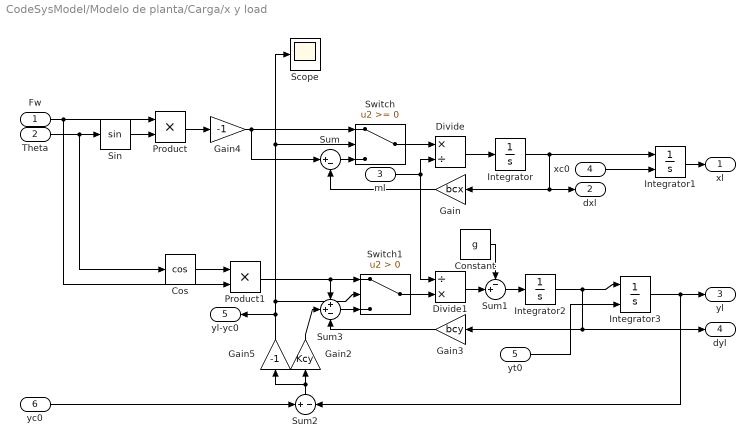
== system CodeSysModel/Modelo de planta/Carga/x y load ==
  Fw : Inport
  Theta : Inport  Port=2
  ml : Inport  Port=3
  xc0 : Inport  Port=4
  yt0 : Inport  Port=5
  yc0 : Inport  Port=6
  Constant : Constant  Value=g
  Cos : Trigonometry  Operator=cos
  Divide : Product  Inputs=*/
  Divide1 : Product  Inputs=/*
  Gain : Gain  Gain=bcx
  Gain2 : Gain  Gain=Kcy
  Gain3 : Gain  Gain=bcy
  Gain4 : Gain  Gain=-1
  Gain5 : Gain  Gain=-1
  Integrator : Integrator  ZeroCross=off
  Integrator1 : Integrator  InitialConditionSource=external  InitialCondition=0.01
  Integrator2 : Integrator
  Integrator3 : Integrator  InitialConditionSource=external  InitialCondition=1
  Product : Product
  Product1 : Product
  Scope : Scope
  Sin : Trigonometry
  Sum : Sum  Inputs=|+-
  Sum1 : Sum  Inputs=-+|
  Sum2 : Sum  Inputs=+-
  Sum3 : Sum  Inputs=++-
  Switch : Switch
  Switch1 : Switch  Criteria=u2 > Threshold
  xl : Outport
  dxl : Outport  Port=2
  yl : Outport  Port=3
  dyl : Outport  Port=4
  yl-yc0 : Outport  Port=5
  wires:
  Fw/1 -> Product/1, Product1/2
  Theta/1 -> Sin/1, Cos/1
  Sin/1 -> Product/2
  Product/1 -> Gain4/1
  Integrator/1 -> dxl/1, Gain/1, Integrator1/1
  Sum/1 -> Switch/3
  Gain/1 -> Sum/2
  Switch/1 -> Divide/1
  Divide/1 -> Integrator/1
  ml/1 -> Divide1/1, Divide/2
  Integrator1/1 -> xl/1
  Cos/1 -> Product1/1
  Product1/1 -> Sum3/1, Switch1/1
  Switch1/1 -> Divide1/2
  Integrator2/1 -> Gain3/1, dyl/1, Integrator3/1
  Integrator3/1 -> yl/1, Sum2/2
  Sum2/1 -> Gain5/1, Gain2/1
  yc0/1 -> Sum2/1
  Sum3/1 -> Switch1/3
  Gain2/1 -> Sum3/2
  Gain3/1 -> Sum3/3
  Gain4/1 -> Sum/1, Switch/1
  Gain5/1 -> yl-yc0/1, Scope/1, Switch/2, Switch1/2
  xc0/1 -> Integrator1/2
  yt0/1 -> Integrator3/2
  ? -> ?
  Constant/1 -> Sum1/1
  Divide1/1 -> Sum1/2
  Sum1/1 -> Integrator2/1

== matlab function CodeSysModel/CurvaPortencia ==
  data: m input; v_Iz_max output
function v_Iz_max  = calc_vmax(m)

p = 956150;

v_Iz_max = p/(m*9.8);

if v_Iz_max>3
    v_Iz_max=3;
    
end

== matlab function CodeSysModel/Algoritmos de busqueda de camino y interpolacion/Astart ==
  data: StartX input; StartY input; x_obj input; OptimalPath2 output size=2,100; y_obj input
function OptimalPath2=ASTARPATH(StartX,StartY,x_obj,y_obj)
%Version 1.0
% By Einar Ueland 2nd of May, 2016
%%%
StartX= round(StartX);
StartY= round(StartY);
dist_seg=2;
MAP=int8(zeros(60,80));
%%% Generating a MAP
%1 represent an object that the path cannot penetrate, zero is a free path
MAP(20,1:30)=1;
MAP(1:20,30)=1;
MAP(80:45,1)=1;
MAP(20:35+dist_seg,30-dist_seg:30+dist_seg)=1;
MAP(20:35+dist_seg,30-dist_seg:30+dist_seg)=1;
MAP(1:30,35)=1;
MAP(1:30,37)=1;
MAP(1:30,39)=1;
MAP(1:30,41)=1;
MAP(1:30,43)=1;
MAP(1:30,45)=1;
MAP(1:30,47)=1;
MAP(1:30,49)=1;
MAP(1:30,51)=1;
MAP(1:30,53)=1;
MAP(1:30,55)=1;

%Start Positions

plot(MAP);
%Generating goal nodes, which is represented by a matrix. Several goals can be speciefied, in which case the pathfinder will find the closest goal. 
%a cell with the value 1 represent a goal cell
GoalRegister=int8(zeros(60,80));
GoalRegister(y_obj,x_obj)=1;
%%%
Connecting_Distance=16;
%nNeighboor=3;
% Preallocation of Matrices
[Height,Width]=size(MAP); %Height and width of matrix
GScore=zeros(Height,Width);           %Matrix keeping track of G-scores 
FScore=single(inf(Height,Width));     %Matrix keeping track of F-scores (only open list) 
Hn=single(zeros(Height,Width));       %Heuristic matrix
OpenMAT=int8(zeros(Height,Width));    %Matrix keeping of open grid cells
ClosedMAT=int8(zeros(Height,Width));  %Matrix keeping track of closed grid cells
ClosedMAT(MAP==1)=1;                  %Adding object-cells to closed matrix
ParentX=zeros(Height,Width);   %Matrix keeping track of X position of parent
ParentY=zeros(Height,Width);   %Matrix keeping track of Y position of parent


%%% Setting up matrices representing neighboors to be investigated
NeighboorCheck=ones(2*Connecting_Distance+1);
Dummy=2*Connecting_Distance+2;
Mid=Connecting_Distance+1;
for i=1:Connecting_Distance-1
NeighboorCheck(i,i)=0;
NeighboorCheck(Dummy-i,i)=0;
NeighboorCheck(i,Dummy-i)=0;
NeighboorCheck(Dummy-i,Dummy-i)=0;
NeighboorCheck(Mid,i)=0;
NeighboorCheck(Mid,Dummy-i)=0;
NeighboorCheck(i,Mid)=0;
NeighboorCheck(Dummy-i,Mid)=0;
end
NeighboorCheck(Mid,Mid)=0;

[row, col]=find(NeighboorCheck==1);
Neighboors=[row col]-(Connecting_Distance+1);
N_Neighboors=size(col,1);
%%% End of setting up matrices representing neighboors to be investigated


%%%%%%%%% Creating Heuristic-matrix based on distance to nearest  goal node
[ row,col]=find(GoalRegister==1);
RegisteredGoals=[row col];
Nodesfound=size(RegisteredGoals,1);

for k=1:size(GoalRegister,1)
    for j=1:size(GoalRegister,2)
        if MAP(k,j)==0
            Mat=RegisteredGoals-(repmat([j k],(Nodesfound),1));
            Distance=(min(sqrt(sum(abs(Mat).^2,2))));
            Hn(k,j)=Distance;
        end
    end
end
%End of creating Heuristic-matrix. 

%Note: If Hn values is set to zero the method will reduce to the Dijkstras method.

%Initializign start node with FValue and opening first node.
FScore(StartY,StartX)=Hn(StartY,StartX);         
OpenMAT(StartY,StartX)=1;   
CurrentY=0;
CurrentX=0;


while 1==1 %Code will break when path found or when no path exist
    MINopenFSCORE=min(min(FScore));
    if MINopenFSCORE==inf;
    %Failuere!
    OptimalPath=[inf];
    RECONSTRUCTPATH=0;
     break
    end
    [CurrentY,CurrentX]=find(FScore==MINopenFSCORE);
    CurrentY=CurrentY(1);
    CurrentX=CurrentX(1);

    if GoalRegister(CurrentY,CurrentX)==1
    %GOAL!!
        RECONSTRUCTPATH=1;
        break
    end
    
  %Remobing node from OpenList to ClosedList  
    OpenMAT(CurrentY,CurrentX)=0;
    FScore(CurrentY,CurrentX)=inf;
    ClosedMAT(CurrentY,CurrentX)=1;
    for p=1:N_Neighboors
        i=Neighboors(p,1); %Y
        j=Neighboors(p,2); %X
        if CurrentY+i<1||CurrentY+i>Height||CurrentX+j<1||CurrentX+j>Width
            continue
        end
        Flag=1;
        if(ClosedMAT(CurrentY+i,CurrentX+j)==0) %Neiboor is open;
            if (abs(i)>1||abs(j)>1);   
                % Need to check that the path does not pass an object
                JumpCells=2*max(abs(i),abs(j))-1;
                for K=1:JumpCells;
                    YPOS=round(K*i/JumpCells);
                    XPOS=round(K*j/JumpCells);
            
                    if (MAP(CurrentY+YPOS,CurrentX+XPOS)==1)
                        Flag=0;
                    end
                end
            end
             %End of  checking that the path does not pass an object

            if Flag==1;           
                tentative_gScore = GScore(CurrentY,CurrentX) + sqrt(i^2+j^2);
                if OpenMAT(CurrentY+i,CurrentX+j)==0
                    OpenMAT(CurrentY+i,CurrentX+j)=1;                    
                elseif tentative_gScore >= GScore(CurrentY+i,CurrentX+j)
                    continue
                end
                ParentX(CurrentY+i,CurrentX+j)=CurrentX;
                ParentY(CurrentY+i,CurrentX+j)=CurrentY;
                GScore(CurrentY+i,CurrentX+j)=tentative_gScore;
                FScore(CurrentY+i,CurrentX+j)= tentative_gScore+Hn(CurrentY+i,CurrentX+j);
            end
        end
    end
end

k=2;
OptimalPath=zeros(100,2);
OptimalPath(:,:)=-1;
if RECONSTRUCTPATH
    OptimalPath(1,:)=[CurrentY CurrentX];
    while RECONSTRUCTPATH
        CurrentXDummy=ParentX(CurrentY,CurrentX);
        CurrentY=ParentY(CurrentY,CurrentX);
        CurrentX=CurrentXDummy;
        OptimalPath(k,:)=[CurrentY CurrentX];
        k=k+1;
        if (((CurrentX== StartX)) &&(CurrentY==StartY))
            break
        end
    end
end
contador=0;
for l=1:100
    if OptimalPath(l,1)~=-1
        contador=contador+1;
    end
end
OptimalPath=OptimalPath';
OptimalPath2=zeros(2,contador);
OptimalPath2=OptimalPath(:,1:contador);

end

== matlab function CodeSysModel/Mode ==
  data: u input; y output
function y = mode(u)
if u==0
y="manual";
elseif u==1
y="automatico";
elseif u==2
y="automatico_simple";
else  
y="automatico_doble";
end

== matlab function CodeSysModel/Position_dump/MATLAB Function ==
  data: qd input size=2,1000000; cont_i input; vt output; vi output
 function [vt,vi] = fcn(qd,cont_i)
 cont_i=int32(cont_i);
 if (cont_i<length(qd(1,:)))
   cont=cont_i+1;
   vt = qd(1,cont);
   vi = qd(2,cont);
 else
  vt = 0;
  vi = 0;
 end
 
 end

== matlab function CodeSysModel/Algoritmos de busqueda de camino y interpolacion/Interpolador ==
  data: wayPoints input size=2,100; q output size=[2,1000000]; velMaxX input; velMaxY input
function q  = Interp(wayPoints,velMaxX,velMaxY)
coder.extrinsic('plot')
pendiente_ant=0;
cont_p=1;
wayPoints=wayPoints([2,1],:);
wayPoints=flip(wayPoints,2);
wayPoints(2,:)=(wayPoints(2,:)-65)*-1;
for i=1:length(wayPoints)-1
    pendiente=(wayPoints(2,i)-wayPoints(2,i+1))/(wayPoints(1,i)-wayPoints(1,i+1));
    if pendiente_ant~=pendiente
        cont_p=cont_p+1;
    end
    pendiente_ant=pendiente;
end
wayPoints1=zeros(2,cont_p);
cont_p2=0;
for i=1:length(wayPoints(1,:))-1
    pendiente=(wayPoints(2,i)-wayPoints(2,i+1))/(wayPoints(1,i)-wayPoints(1,i+1));
    if pendiente_ant~=pendiente
    cont_p2=cont_p2+1;
    wayPoints1(:,cont_p2)=wayPoints(:,i);
    end
    pendiente_ant=pendiente;
end
wayPoints1(:,end)=wayPoints(:,end);
wayPoints1(:,1)=wayPoints(:,1);
figure(10)
plot(wayPoints1(1,:),wayPoints1(2,:))   
vx_max=velMaxX;
vy_max=velMaxY;
timePoints1=zeros(1,length(wayPoints1));
tiempo_ant=0;
for i=1:length(wayPoints1(1,:))-1
    restaX=abs(wayPoints1(1,i+1)-wayPoints1(1,i));
    restaY=abs(wayPoints1(2,i+1)-wayPoints1(2,i));
    timex=restaX/(vx_max/2.5);
    timey=restaY/(vy_max/2.5);
    if timex>timey
    timePoints1(i+1)=restaX/(vx_max/4)+tiempo_ant;
    elseif timex<timey
    timePoints1(i+1)=restaY/(vy_max/4)+tiempo_ant;
    else
     timePoints1(i+1)=restaX/(vx_max/4)+tiempo_ant;    
    end
    tiempo_ant=timePoints1(i+1);
end
tSamples1=0:2e-2:timePoints1(end);
q = zeros(2,length(tSamples1));%'VelocityBoundaryCondition',vel_max);
qx=interp1(timePoints1,wayPoints1(1,:),tSamples1,'pchip');
qy=interp1(timePoints1,wayPoints1(2,:),tSamples1,'pchip');
q(1,:)=qx;
q(2,:)=qy;
figure(15)
plot(qx,qy)  

end
